simulink model "vehicle_dynamic_dis_3states"  (R2022b)
settings: Solver=VariableStepAuto  StartTime=0.0  StopTime=120  RelTol=1e-3
values from neighbouring files (symbols this model uses):
  B_full = B * Ts    [vehicle_lateral_control_LMIs_3states_auto.m]
  C_dis = V_DIS.C    [vehicle_lateral_control_LMIs.m]    (also in vehicle_lateral_control_LMIs_3states.m; vehicle_lateral_control_LMIs_3states_auto.m)
  Cf = 57117    [vehicle_lateral_control_LMIs.m]    (also in vehicle_lateral_control_LMIs_3states.m; vehicle_lateral_control_LMIs_3states_auto.m)
  Cr = 81396    [vehicle_lateral_control_LMIs.m]    (also in vehicle_lateral_control_LMIs_3states.m; vehicle_lateral_control_LMIs_3states_auto.m)
  D_dis = V_DIS.D    [vehicle_lateral_control_LMIs.m]    (also in vehicle_lateral_control_LMIs_3states.m; vehicle_lateral_control_LMIs_3states_auto.m)
  Iz = 1975    [vehicle_lateral_control_LMIs.m]    (also in vehicle_lateral_control_LMIs_3states.m; vehicle_lateral_control_LMIs_3states_auto.m)
  K_gain = K_lmi    [vehicle_lateral_control_LMIs.m]    (also in vehicle_lateral_control_LMIs_3states.m = K_dlqr; vehicle_lateral_control_LMIs_3states_auto.m = K_dlqr)
  Ka = value(Ya)*inv(value(P))    [vehicle_lateral_control_LMIs_3states_auto.m]
  Kb = value(Yb)*inv(value(P))    [vehicle_lateral_control_LMIs_3states_auto.m]
  Kc = value(Yc)*inv(value(P))    [vehicle_lateral_control_LMIs_3states_auto.m]
  lf = 1.15    [vehicle_lateral_control_LMIs.m]    (also in vehicle_lateral_control_LMIs_3states.m; vehicle_lateral_control_LMIs_3states_auto.m)
  lr = 1.38    [vehicle_lateral_control_LMIs.m]    (also in vehicle_lateral_control_LMIs_3states.m; vehicle_lateral_control_LMIs_3states_auto.m)
  m = 1621    [vehicle_lateral_control_LMIs.m]    (also in vehicle_lateral_control_LMIs_3states.m; vehicle_lateral_control_LMIs_3states_auto.m)
  Ts = 0.01    [trajectory_test.m]    (also in vehicle_lateral_control_LMIs.m = 0.009; vehicle_lateral_control_LMIs_3states.m; vehicle_lateral_control_LMIs_3states_auto.m)
  vx = 0    [trajectory_test.m]    (also in vehicle_lateral_control_LMIs.m = 20; vehicle_lateral_control_LMIs_3states.m = 20; vehicle_lateral_control_LMIs_3states_auto.m = 15)
  vx_track = 5    [vehicle_lateral_control_LMIs_3states.m]    (also in vehicle_lateral_control_LMIs_3states_auto.m)
  wp = wpt(L,vx_ref)    [trajectory_test_2.m]    (also in vehicle_lateral_control_LMIs_3states.m = wpt(L,vx_track); vehicle_lateral_control_LMIs_3states_auto.m = wpt(L,vx_track))
libraries: cstblocks x1
settings Model: Creator=phatdo  LastModifiedBy=phatdo
settings DataIOCC: ReturnWorkspaceOutputs=off

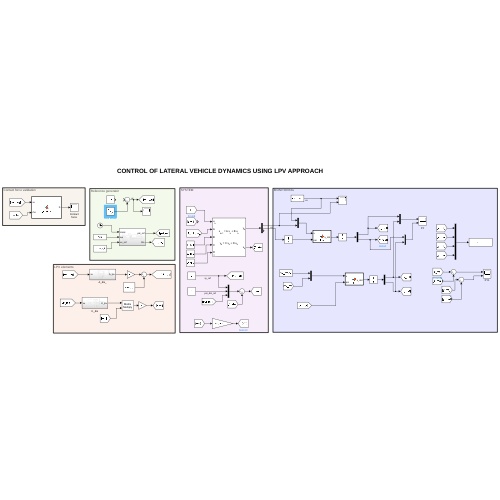
[thumbnail: Simulink's stored preview of the top-level diagram]
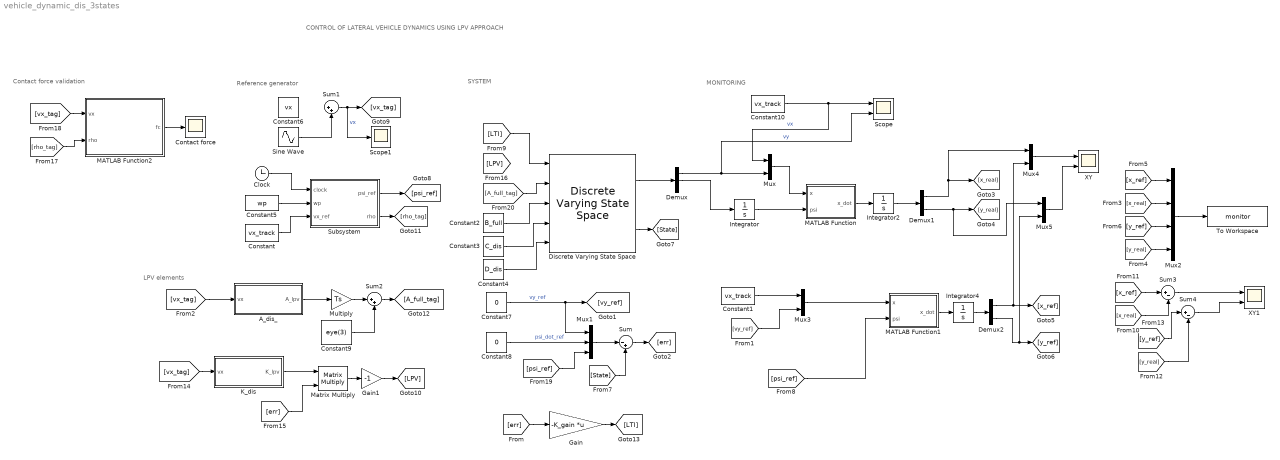
== system vehicle_dynamic_dis_3states ==
  note: CONTROL OF LATERAL VEHICLE DYNAMICS USING LPV APPROACH
  note: SYSTEM
  note: LPV elements
  note: Reference generator
  note: Contact force validation
  note: MONITORING
  A_dis_ : Subsystem
  Clock : Clock
  Constant : Constant  Value=vx_track
  Constant1 : Constant  Value=vx_track
  Constant10 : Constant  Value=vx_track
  Constant2 : Constant  Value=B_full
  Constant3 : Constant  Value=C_dis
  Constant4 : Constant  Value=D_dis
  Constant5 : Constant  Value=wp
  Constant6 : Constant  Value=vx
  Constant7 : Constant  Value=0
  Constant8 : Constant  Value=0
  Constant9 : Constant  Value=eye(3)
  Contact force : Scope
  Demux : Demux  Outputs=3
  Demux1 : Demux  Outputs=2
  Demux2 : Demux  Outputs=2
  Discrete Varying State Space : cstblocks/Linear Parameter Varying/Discrete Varying State Space  x0=0  Ts=Ts  OutputX=on  OutputDX=off
  Gain : Gain  Gain=-K_gain  Multiplication=Matrix(K*u) (u vector)
  Gain1 : Gain  Gain=-1
  Integrator : Integrator
  Integrator2 : Integrator
  Integrator4 : Integrator
  K_dis : Subsystem
  MATLAB Function : MATLAB Function  TreatAsAtomicUnit=on
  MATLAB Function1 : MATLAB Function  TreatAsAtomicUnit=on
  MATLAB Function2 : MATLAB Function  TreatAsAtomicUnit=on
  Matrix Multiply : Product  Multiplication=Matrix(*)
  Multiply : Gain  Gain=Ts
  Mux{,3..5} (4 alike) : Mux  Inputs=2
  Mux1 : Mux  Inputs=3
  Mux2 : Mux
  Scope : Scope  NumInputPorts=2
  Scope1 : Scope
  Sine Wave : Sin  Amplitude=3  Bias=15  SampleTime=0
  Subsystem : Subsystem
  Sum : Sum  Inputs=|-+
  Sum1 : Sum  Inputs=|++
  Sum2 : Sum  Inputs=|++
  Sum3 : Sum  Inputs=|+-
  Sum4 : Sum  Inputs=|+-
  To Workspace : ToWorkspace  VariableName=monitor  SaveFormat=Timeseries  SampleTime=-1
  XY : Scope  NumInputPorts=2
  XY1 : Scope  NumInputPorts=2
  wires:
  Discrete Varying State Space/1 -> Demux/1
  Demux/1 -> Scope/2, Mux/2  "vy"
  Mux/1 -> MATLAB Function/1(x)
  Demux/2 -> Integrator/1
  Integrator/1 -> MATLAB Function/2(psi)
  MATLAB Function/1(x_dot) -> Integrator2/1
  Integrator2/1 -> Demux1/1
  Sum/1 -> [err]
  Mux1/1 -> Sum/1
  Constant7/1 -> [vy_ref], Mux1/1  "vy_ref"
  [vy_ref] -> Mux3/2
  Mux3/1 -> MATLAB Function1/1(x)
  MATLAB Function1/1(x_dot) -> Integrator4/1
  Integrator4/1 -> Demux2/1
  Constant1/1 -> Mux3/1
  [psi_ref] -> MATLAB Function1/2(psi)
  Demux1/1 -> [x_real], Mux4/1
  Demux1/2 -> Mux5/1, [y_real]
  Demux2/1 -> Mux4/2, [x_ref]
  Demux2/2 -> Mux5/2, [y_ref]
  [x_ref] -> Mux2/1
  [x_real] -> Mux2/2
  [y_ref] -> Mux2/3
  [y_real] -> Mux2/4
  Mux2/1 -> To Workspace/1
  Mux4/1 -> XY/1
  Constant8/1 -> Mux1/2  "psi_dot_ref"
  Constant2/1 -> Discrete Varying State Space/3
  Constant3/1 -> Discrete Varying State Space/4
  Constant4/1 -> Discrete Varying State Space/5
  Discrete Varying State Space/2 -> [State]
  [State] -> Sum/2
  Mux5/1 -> XY/2
  Constant5/1 -> Subsystem/2(wp)
  Clock/1 -> Subsystem/1(clock)
  Constant/1 -> Subsystem/3(vx_ref)
  Sum1/1 -> Scope1/1, [vx_tag]  "vx"
  [vx_tag] -> A_dis_/1(vx)
  A_dis_/1(A_lpv) -> Multiply/1
  Multiply/1 -> Sum2/1
  Constant9/1 -> Sum2/2
  Subsystem/1(psi_ref) -> [psi_ref]
  Sum3/1 -> XY1/1
  Sum4/1 -> XY1/2
  [x_ref] -> Sum3/1
  [x_real] -> Sum3/2
  [y_ref] -> Sum4/1
  [y_real] -> Sum4/2
  K_dis/1(K_lpv) -> Matrix Multiply/1
  [vx_tag] -> K_dis/1(vx)
  [err] -> Matrix Multiply/2
  Matrix Multiply/1 -> Gain1/1
  Gain1/1 -> [LPV]
  Subsystem/2(rho) -> [rho_tag]
  [rho_tag] -> MATLAB Function2/2(rho)
  MATLAB Function2/1(fc) -> Contact force/1
  [vx_tag] -> MATLAB Function2/1(vx)
  [psi_ref] -> Mux1/3
  Sum2/1 -> [A_full_tag]
  [A_full_tag] -> Discrete Varying State Space/2
  Constant10/1 -> Scope/1, Mux/1  "vx"
  [err] -> Gain/1
  Gain/1 -> [LTI]
  Sine Wave/1 -> Sum1/2
  [LTI] -> Discrete Varying State Space/1

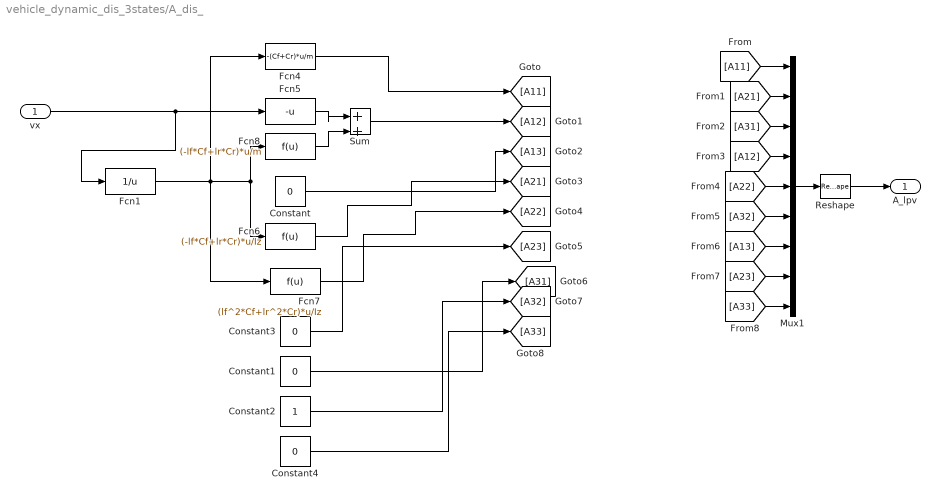
== system vehicle_dynamic_dis_3states/A_dis_ ==
  vx : Inport
  Constant{,1,3..4} (4 alike) : Constant  Value=0
  Constant2 : Constant
  Fcn1 : Fcn  Expr=1/u
  Fcn4 : Fcn  Expr=-(Cf+Cr)*u/m
  Fcn5 : Fcn  Expr=-u
  Fcn6 : Fcn  Expr=(-lf*Cf+lr*Cr)*u/Iz
  Fcn7 : Fcn  Expr=(lf^2*Cf+lr^2*Cr)*u/Iz
  Fcn8 : Fcn  Expr=(-lf*Cf+lr*Cr)*u/m
  Mux1 : Mux  Inputs=9
  Reshape : Reshape  OutputDimensionality=Customize  OutputDimensions=[3;3]
  Sum : Sum  Inputs=|++
  A_lpv : Outport
  wires:
  Reshape/1 -> A_lpv/1
  Fcn4/1 -> [A11]
  Fcn1/1 -> Fcn6/1, Fcn8/1, Fcn7/1, Fcn4/1
  Fcn5/1 -> Sum/1
  Fcn8/1 -> Sum/2
  Sum/1 -> [A12]
  vx/1 -> Fcn1/1, Fcn5/1
  Constant/1 -> [A13]
  Fcn6/1 -> [A21]
  Fcn7/1 -> [A22]
  Constant3/1 -> [A23]
  Constant1/1 -> [A31]
  Constant2/1 -> [A32]
  Constant4/1 -> [A33]
  Mux1/1 -> Reshape/1
  [A11] -> Mux1/1
  [A21] -> Mux1/2
  [A31] -> Mux1/3
  [A12] -> Mux1/4
  [A22] -> Mux1/5
  [A32] -> Mux1/6
  [A13] -> Mux1/7
  [A23] -> Mux1/8
  [A33] -> Mux1/9

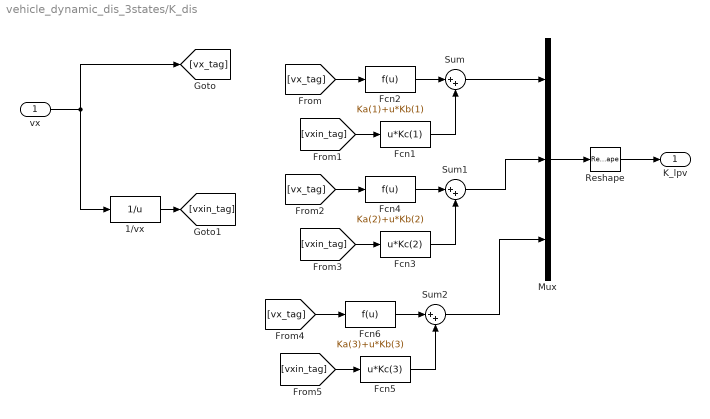
== system vehicle_dynamic_dis_3states/K_dis ==
  vx : Inport
  1/vx : Fcn  Expr=1/u
  Fcn1 : Fcn  Expr=u*Kc(1)
  Fcn2 : Fcn  Expr=Ka(1)+u*Kb(1)
  Fcn3 : Fcn  Expr=u*Kc(2)
  Fcn4 : Fcn  Expr=Ka(2)+u*Kb(2)
  Fcn5 : Fcn  Expr=u*Kc(3)
  Fcn6 : Fcn  Expr=Ka(3)+u*Kb(3)
  Mux : Mux  Inputs=3
  Reshape : Reshape  OutputDimensionality=Customize  OutputDimensions=[1,3]
  Sum : Sum  Inputs=|++
  Sum1 : Sum  Inputs=|++
  Sum2 : Sum  Inputs=|++
  K_lpv : Outport
  wires:
  Mux/1 -> Reshape/1
  Reshape/1 -> K_lpv/1
  vx/1 -> [vx_tag], 1/vx/1
  Fcn2/1 -> Sum/1
  Sum/1 -> Mux/1
  [vx_tag] -> Fcn2/1
  1/vx/1 -> [vxin_tag]
  [vxin_tag] -> Fcn1/1
  Fcn1/1 -> Sum/2
  [vx_tag] -> Fcn4/1
  Fcn3/1 -> Sum1/2
  Sum1/1 -> Mux/2
  Fcn4/1 -> Sum1/1
  [vxin_tag] -> Fcn3/1
  Fcn5/1 -> Sum2/2
  [vx_tag] -> Fcn6/1
  [vxin_tag] -> Fcn5/1
  Fcn6/1 -> Sum2/1
  Sum2/1 -> Mux/3

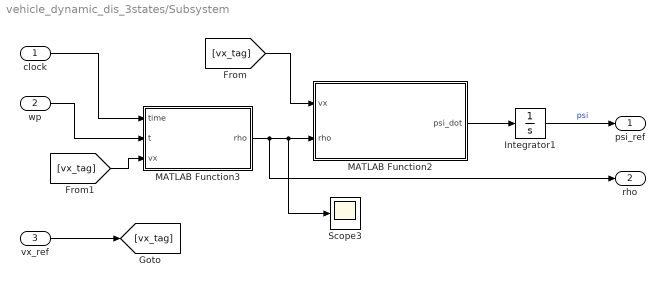
== system vehicle_dynamic_dis_3states/Subsystem ==
  clock : Inport
  wp : Inport  Port=2
  vx_ref : Inport  Port=3
  Integrator1 : Integrator
  MATLAB Function2 : MATLAB Function  TreatAsAtomicUnit=on
  MATLAB Function3 : MATLAB Function  TreatAsAtomicUnit=on
  Scope3 : Scope
  psi_ref : Outport
  rho : Outport  Port=2
  wires:
  MATLAB Function2/1(psi_dot) -> Integrator1/1
  MATLAB Function3/1(rho) -> rho/1, Scope3/1, MATLAB Function2/2(rho)
  clock/1 -> MATLAB Function3/1(time)
  wp/1 -> MATLAB Function3/2(t)
  Integrator1/1 -> psi_ref/1  "psi"
  vx_ref/1 -> [vx_tag]
  [vx_tag] -> MATLAB Function2/1(vx)
  [vx_tag] -> MATLAB Function3/3(vx)

== matlab function vehicle_dynamic_dis_3states/MATLAB Function ==
  data: x input; x_dot output; psi input
function x_dot = fcn(x, psi)

% x = [vx, vy]

x_dot = zeros(2,1);

vx = x(1);
vy = x(2);

x_dot(1) = vx*cos(psi) - vy*sin(psi);
x_dot(2) = vx*sin(psi) + vy*cos(psi);

end

== matlab function vehicle_dynamic_dis_3states/Subsystem/MATLAB Function2 ==
  data: vx input; psi_dot output; rho input
function psi_dot = yawrate(vx, rho)
    psi_dot = rho*vx; % Yaw rate
end

== matlab function vehicle_dynamic_dis_3states/MATLAB Function1 ==
  data: x input; x_dot output; psi input
function x_dot = fcn(x, psi)

% x = [vx, vy]

x_dot = zeros(2,1);

vx = x(1);
vy = x(2);

x_dot(1) = vx*cos(psi) - vy*sin(psi);
x_dot(2) = vx*sin(psi) + vy*cos(psi);

end

== matlab function vehicle_dynamic_dis_3states/Subsystem/MATLAB Function3 ==
  data: time input; t input; rho output; vx input
function rho = track_generator(time,t,vx)


rho = 0;
clothoide_const = 3600;
R = 0;
vx = 5;

if time >= t(1) && time < t(2) 
    rho = 0;% go straight
elseif time >= t(2) && time < t(3)
    rho = -vx*(time - t(2))/clothoide_const; % clothoide cornering
elseif time >= t(3) && time < t(4)
%     rho = -1/R; % circle cornering
      rho = -vx*(t(3) - t(2))/clothoide_const; % circle cornering
elseif time >= t(4) && time < t(5)
    rho = 0;% go straight
elseif time >= t(5) && time < t(6)
    rho = -vx*(time - t(5))/clothoide_const; % clothoide cornering
elseif time >= t(6) && time < t(7)
    rho = -vx*(t(6) - t(5))/clothoide_const; % circle cornering
elseif time >= t(7) && time < t(8)
    rho = 0;
elseif time >= t(8) && time < t(9)
    rho = vx*(time - t(8))/clothoide_const; % clothoide cornering
elseif time >= t(9) && time < t(10)
    rho = vx*(t(9) - t(8))/clothoide_const; % circle cornering
else
    rho = 0;
end


end

== matlab function vehicle_dynamic_dis_3states/MATLAB Function2 ==
  data: vx input; fc output; rho input
function fc = F_contact(vx,rho)

m = 1621;

fc = m*vx^2*rho;
end
